simulink model "consigna_torque"  (R2020a)
settings: Solver=VariableStepAuto  StartTime=0.0  StopTime=10.0  RelTol=1e-3
model workspace: external: MATLAB File D:\Ferran\Facultad\UNCuyo\Meca\Automática y Máquinas Eléctricas\Proyecto final\matlab2\parametros_y_especs\parametros_y_especif.m (data not in the file)
undefined symbols (not defined in the file): beq, lambda_m, Ld, Lq, Pp
settings Model: Creator=Ferran  LastModifiedBy=Ferran

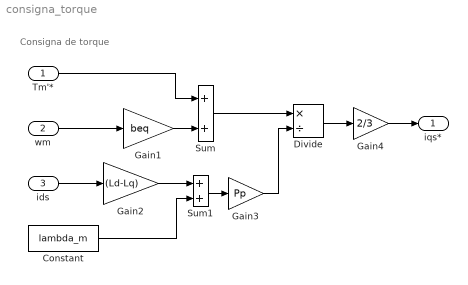
== system consigna_torque ==
  note: Consigna de torque
  Tm'* : Inport
  wm : Inport  Port=2
  ids : Inport  Port=3
  Constant : Constant  Value=lambda_m
  Divide : Product  Inputs=*/
  Gain1 : Gain  Gain=beq
  Gain2 : Gain  Gain=(Ld-Lq)
  Gain3 : Gain  Gain=Pp
  Gain4 : Gain  Gain=2/3
  Sum : Sum
  Sum1 : Sum
  iqs* : Outport
  wires:
  wm/1 -> Gain1/1
  Gain1/1 -> Sum/2
  Tm'*/1 -> Sum/1
  ids/1 -> Gain2/1
  Constant/1 -> Sum1/2
  Gain2/1 -> Sum1/1
  Sum/1 -> Divide/1
  Sum1/1 -> Gain3/1
  Gain3/1 -> Divide/2
  Divide/1 -> Gain4/1
  Gain4/1 -> iqs*/1
